simulink model "simulacao_sem_linearizar3"  (R2017a)
settings: Solver=VariableStepAuto  StartTime=0.0  StopTime=30  RelTol=1e-3
values from neighbouring files (symbols this model uses):
  a = -9128    [prepare_y_prbs.m]
undefined symbols (not defined in the file or in its folder): g, m
settings Model: Creator=Mateus  LastModifiedBy=mateu

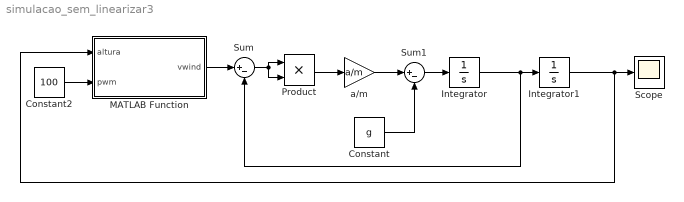
== system simulacao_sem_linearizar3 ==
  Constant : Constant  Value=g
  Constant2 : Constant  Value=100
  Integrator : Integrator
  Integrator1 : Integrator
  MATLAB Function : MATLAB Function  TreatAsAtomicUnit=on
  Product : Product
  Scope : Scope
  Sum : Sum  Inputs=|+-
  Sum1 : Sum  Inputs=|+-
  a/m : Gain  Gain=a/m
  wires:
  Integrator/1 -> Sum/2, Integrator1/1
  Sum/1 -> Product/1, Product/2
  Product/1 -> a/m/1
  a/m/1 -> Sum1/1
  Sum1/1 -> Integrator/1
  Constant/1 -> Sum1/2
  Constant2/1 -> MATLAB Function/2(pwm)
  Integrator1/1 -> MATLAB Function/1(altura), Scope/1
  MATLAB Function/1(vwind) -> Sum/1

== matlab function simulacao_sem_linearizar3/MATLAB Function ==
  data: altura input; vwind output; pwm input
function vwind = fittedmodel(altura,pwm)

p00 =       18.37;
p10 =     -0.5502;
p01 =       0.224;
p20 =      0.0105;
p11 =   -0.003002;
p02 =  -0.0006906;
p30 =  -6.885e-05;
p21 =   1.084e-05;
p12 =   8.743e-06;
p03 =   2.752e-07;
vwind = p00 + p10*altura + p01*pwm + p20*altura^2 + p11*altura*pwm + p02*pwm^2 + p30*altura^3 + p21*altura^2*pwm + p12*altura*pwm^2 + p03*pwm^3;
if vwind <0 
    vwind=0;
end

end
